simulink model "SensorSignals"  (R2024b)
settings: Solver=FixedStepAuto  StartTime=0.0  StopTime=10.0  RelTol=1e-3
settings Model: DataDictionary=Master_Dictionary.sldd  EnableAccessToBaseWorkspace=off  Creator=torni  LastModifiedBy=will
settings SolverCC: AlgebraicLoopSolver=TrustRegion
settings DataIOCC: ReturnWorkspaceOutputs=off
settings OptimizationCC: DefaultParameterBehavior=Inlined  EnhancedBackFolding=on  PassReuseOutputArgsAs=Individual arguments  ZeroExternalMemoryAtStartup=off  ZeroInternalMemoryAtStartup=off  OptimizeBlockOrder=speed  DifferentSizesBufferReuse=on  OptimizationCustomize=off  EfficientTunableParamExpr=on
settings DebuggingCC: ParameterTunabilityLossMsg=error  UnconnectedInputMsg=warning  UnconnectedOutputMsg=warning  UnconnectedLineMsg=warning  ArithmeticOperatorsInVariantConditions=warning
settings HardwareCC: TargetLargestAtomicInteger=Long  TargetLargestAtomicFloat=Double  TargetIntDivRoundTo=Zero  TargetEndianess=LittleEndian  TargetHWDeviceType=ARM Compatible->ARM Cortex-M  ProdEqTarget=off
settings ModelReferenceCC: EnableRefExpFcnMdlSchedulingChecks=on
settings SFSimCC: MATLABDynamicMemAlloc=off  CustomCodeUndefinedFunction=UseInterfaceOnly
settings RTWCC: Description=Embedded Coder  SystemTargetFile=ert.tlc  TemplateMakefile=ert_default_tmf  Toolchain=GNU Tools for ARM Embedded Processors  RTWCompilerOptimization=on  GPUComputeCapability=3.5
settings CodeAppCC: ForceParamTrailComments=on  IgnoreCustomStorageClasses=off  OperatorAnnotations=on  SimulinkDataObjDesc=on  SFDataObjDesc=on  InsertBlockDesc=on
settings ERTTargetCC: TargetLangStandard=C99 (ISO)  GenerateSampleERTMain=on  ERTCustomFileTemplate=example_file_process.tlc

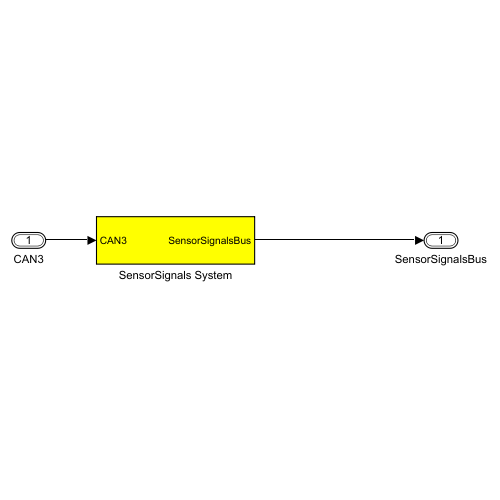
[thumbnail: Simulink's stored preview of the top-level diagram]
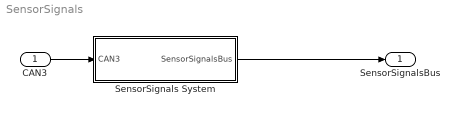
== system SensorSignals ==
  CAN3 : Inport  OutDataTypeStr=Bus: CAN3Bus
  SensorSignals System : Subsystem
  SensorSignalsBus : Outport  OutDataTypeStr=Bus: SensorSignalsBus  VectorParamsAs1DForOutWhenUnconnected=off
  wires:
  CAN3/1 -> SensorSignals System/1(CAN3)
  SensorSignals System/1(SensorSignalsBus) -> SensorSignalsBus/1

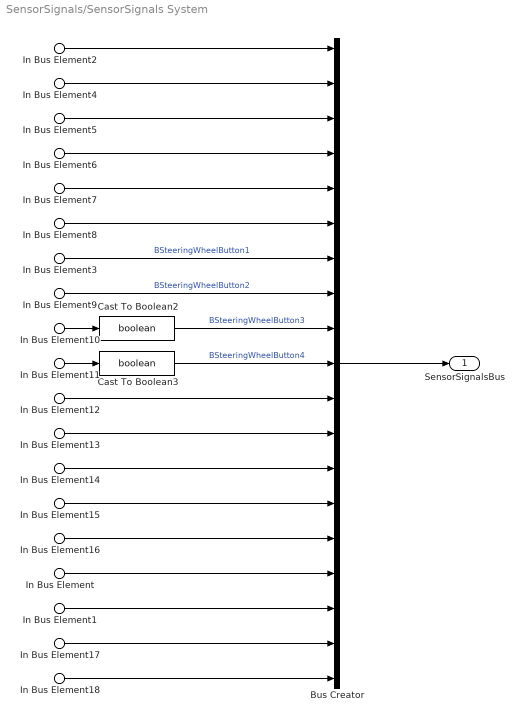
== system SensorSignals/SensorSignals System ==
  In Bus Element : Inport  PortName=CAN3  Element=DDU7Bus.VBrakeF
  In Bus Element1 : Inport  PortName=CAN3  Element=DDU7Bus.VBrakeR
  In Bus Element2 : Inport  PortName=CAN3  Element=DDU7Bus.VDamperPotentiometerFL
  In Bus Element4 : Inport  PortName=CAN3  Element=DDU7Bus.VDamperPotentiometerFR
  In Bus Element5 : Inport  PortName=CAN3  Element=DDU7Bus.NDisplayNumberDDU7
  In Bus Element6 : Inport  PortName=CAN3  Element=DDU7Bus.VSteeringAngle
  In Bus Element7 : Inport  PortName=CAN3  Element=DDU7Bus.VThrottlePedal1
  In Bus Element8 : Inport  PortName=CAN3  Element=DDU7Bus.VThrottlePedal2
  In Bus Element17 : Inport  PortName=CAN3  Element=DDU7Bus.VDamperPotentiometerRL
  In Bus Element18 : Inport  PortName=CAN3  Element=DDU7Bus.VDamperPotentiometerRR
  In Bus Element3 : Inport  PortName=CAN3  Element=SteeringWheelBus.BSteeringWheelButton1
  In Bus Element9 : Inport  PortName=CAN3  Element=SteeringWheelBus.BSteeringWheelButton2
  In Bus Element10 : Inport  PortName=CAN3  Element=SteeringWheelBus.BSteeringWheelButton3
  In Bus Element11 : Inport  PortName=CAN3  Element=SteeringWheelBus.BSteeringWheelButton4
  In Bus Element12 : Inport  PortName=CAN3  Element=SteeringWheelBus.NPageSelectRotary
  In Bus Element13 : Inport  PortName=CAN3  Element=SteeringWheelBus.NParameterRotary
  In Bus Element14 : Inport  PortName=CAN3  Element=SteeringWheelBus.NEventModeRotary
  In Bus Element15 : Inport  PortName=CAN3  Element=SteeringWheelBus.VRegenPaddle1
  In Bus Element16 : Inport  PortName=CAN3  Element=SteeringWheelBus.VRegenPaddle2
  Bus Creator : BusCreator  Inputs=19  OutDataTypeStr=Bus: SensorSignalsBus  NonVirtualBus=on
  Cast To Boolean2 : DataTypeConversion  OutDataTypeStr=boolean  SaturateOnIntegerOverflow=off  RndMeth=Floor
  Cast To Boolean3 : DataTypeConversion  OutDataTypeStr=boolean  SaturateOnIntegerOverflow=off  RndMeth=Floor
  SensorSignalsBus : Outport  OutDataTypeStr=Bus: SensorSignalsBus  VectorParamsAs1DForOutWhenUnconnected=off  LockScale=on
  wires:
  In Bus Element2/1 -> Bus Creator/1
  In Bus Element5/1 -> Bus Creator/3
  In Bus Element6/1 -> Bus Creator/4
  In Bus Element7/1 -> Bus Creator/5
  In Bus Element8/1 -> Bus Creator/6
  In Bus Element10/1 -> Cast To Boolean2/1
  In Bus Element11/1 -> Cast To Boolean3/1
  In Bus Element12/1 -> Bus Creator/11
  In Bus Element13/1 -> Bus Creator/12
  In Bus Element14/1 -> Bus Creator/13
  In Bus Element15/1 -> Bus Creator/14
  In Bus Element16/1 -> Bus Creator/15
  In Bus Element/1 -> Bus Creator/16
  In Bus Element1/1 -> Bus Creator/17
  Bus Creator/1 -> SensorSignalsBus/1
  In Bus Element4/1 -> Bus Creator/2
  In Bus Element17/1 -> Bus Creator/18
  In Bus Element18/1 -> Bus Creator/19
  In Bus Element3/1 -> Bus Creator/7  "BSteeringWheelButton1"
  In Bus Element9/1 -> Bus Creator/8  "BSteeringWheelButton2"
  Cast To Boolean2/1 -> Bus Creator/9  "BSteeringWheelButton3"
  Cast To Boolean3/1 -> Bus Creator/10  "BSteeringWheelButton4"
